simulink model "Exa_1"  (R2015a)
settings: Solver=ode23tb  StartTime=0.0  StopTime=15
settings Model: Creator=victo  LastModifiedBy=victo

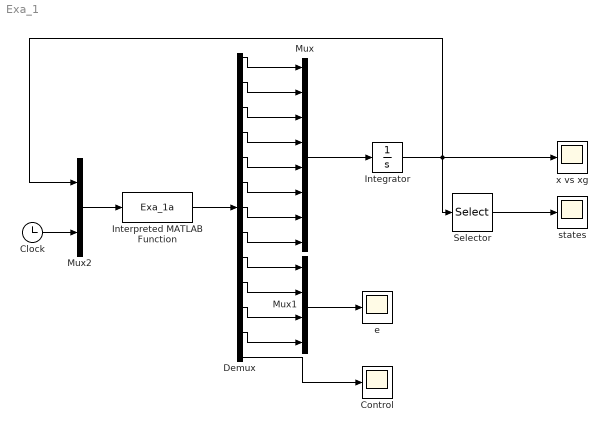
== system Exa_1 ==
  Clock : Clock
  Control : Scope
      settings: TimeRange=15  YMin=3752  YMax=3769  SaveName=Control
  Demux : Demux  Outputs=13
  Integrator : Integrator  InitialCondition=[-1.2 0.5 0.7 -0.6 0 0.0 0.0 0.0]'
  Interpreted MATLAB Function : MATLABFcn  MATLABFcn=Exa_1a  OutputDimensions=13
  Mux : Mux  Inputs=8
  Mux1 : Mux
  Mux2 : Mux  Inputs=2
  Selector : Selector  InputPortWidth=8  Indices=[1:4]
  e : Scope
      settings: SaveName=error
  states : Scope
      settings: YMin=-0.25  YMax=0.325  SaveName=estados
  x vs xg : Scope
      settings: YMin=-15  YMax=15
  wires:
  Integrator/1 -> Selector/1, Mux2/1, x vs xg/1
  Interpreted MATLAB Function/1 -> Demux/1
  Mux/1 -> Integrator/1
  Demux/10 -> Mux1/2
  Demux/12 -> Mux1/4
  Demux/11 -> Mux1/3
  Demux/9 -> Mux1/1
  Mux1/1 -> e/1
  Demux/2 -> Mux/2
  Demux/3 -> Mux/3
  Demux/4 -> Mux/4
  Demux/5 -> Mux/5
  Demux/1 -> Mux/1
  Demux/6 -> Mux/6
  Demux/7 -> Mux/7
  Demux/8 -> Mux/8
  Mux2/1 -> Interpreted MATLAB Function/1
  Clock/1 -> Mux2/2
  Demux/13 -> Control/1
  Selector/1 -> states/1
